simulink model "Optimized_Architecture"  (R2015b)
settings: Solver=FixedStepDiscrete  SolverMode=SingleTasking  StartTime=0.0  StopTime=1000e-6  RelTol=1e-3
libraries: shlslibv1 x282
(part 2 of 2)

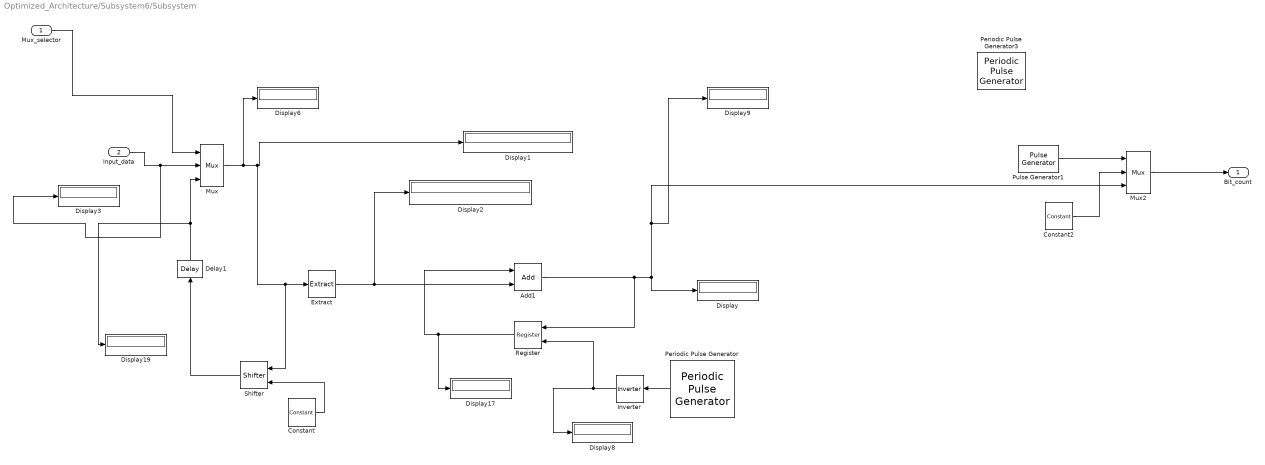
== system Optimized_Architecture/Subsystem6/Subsystem ==
  Mux_selector : Inport
  Input_data : Inport  Port=2
  Add1 : shlslibv1/Math Functions/Add  syn_add_opr=++  syn_out_f=Specify  syn_out_wl=10  syn_out_fl=0  syn_out_dt=unsigned  syn_out_sat=off  syn_out_rnd=Floor (Truncate)  synBlockType=primitive  synLatency=0  synBlockId=96  syn_sum_of_rows=off  syn_inh_port=off  syn_inh_st=on  syn_inh_stf=1  syn_en_pipe=off  syn_pipe_stg=10  syn_flow_ctrl=off
  Constant : shlslibv1/Sources/Constant  syn_cst_val=1  syn_cst_format=Automatic  syn_cst_wl=1  syn_cst_fl=0  syn_cst_dt=unsigned  syn_cst_rnd=on  syn_cst_st=-1  synBlockType=primitive  synLatency=0  synBlockId=15
  Constant2 : shlslibv1/Sources/Constant  syn_cst_val=0  syn_cst_format=Automatic  syn_cst_wl=1  syn_cst_fl=0  syn_cst_dt=unsigned  syn_cst_rnd=on  syn_cst_st=-1  synBlockType=primitive  synLatency=0  synBlockId=15
  Delay1 : shlslibv1/Memories/Delay  syn_delay_val=30  synBlockType=primitive  synLatency=30  synBlockId=104
  Display{,1..3,6,8..9,17,19} (9 alike) : Display
      Display settings: Format=decimal (Stored Integer)
      Display1 settings: Format=binary (Stored Integer)
      Display17 settings: Format=decimal (Stored Integer)
      Display19 settings: Format=decimal (Stored Integer)
      Display2 settings: Format=binary (Stored Integer)
      Display3 settings: Format=decimal (Stored Integer)
      Display8 settings: Format=decimal (Stored Integer)
      Display9 settings: Format=decimal (Stored Integer)
  Extract : shlslibv1/Signal Operations/Extract  syn_extract_vec=0  synBlockType=primitive  synLatency=0  synBlockId=17
  Inverter : shlslibv1/Math Functions/Inverter  syn_out_f=Automatic  syn_out_wl=16  syn_out_fl=8  syn_out_dt=signed  synBlockType=primitive  synLatency=0  synBlockId=10
  Mux : shlslibv1/Signal Operations/Mux  syn_in_nb=2  syn_out_f=Specify  syn_out_wl=10  syn_out_fl=0  syn_out_dt=unsigned  syn_en_se=off  synBlockType=primitive  synLatency=0  synBlockId=16
  Mux2 : shlslibv1/Signal Operations/Mux  syn_in_nb=2  syn_out_f=Specify  syn_out_wl=10  syn_out_fl=0  syn_out_dt=unsigned  syn_en_se=off  synBlockType=primitive  synLatency=0  synBlockId=16
  Periodic Pulse Generator : shlslibv1/Sources/Periodic Pulse  Generator  syn_period_type=Constant  syn_period=309  syn_pw_type=Constant  syn_pw=307  syn_pd_type=Constant  syn_pd=0  syn_en_port=off  syn_st=1/1e6  synBlockType=custom  synLatency=0
  Periodic Pulse Generator3 : shlslibv1/Sources/Periodic Pulse  Generator  syn_period_type=Constant  syn_period=312  syn_pw_type=Constant  syn_pw=31  syn_pd_type=Constant  syn_pd=0  syn_en_port=off  syn_st=1/1e6  synBlockType=custom  synLatency=0
  Pulse Generator1 : shlslibv1/Sources/Pulse Generator  syn_siggentype=Step (0 to 1)  syn_usectl=off  syn_trigedge=rising  syn_triginit=low  syn_stpdel=271  syn_impwidth=1  syn_impdel=1  syn_st=1/1e6  synBlockType=custom  synLatency=0
  Register : shlslibv1/Memories/Register  syn_delay_val=30  syn_rst_val=All zeros  syn_rst_vec=5  syn_rst_port=on  syn_en_port=off  synBlockType=custom  synLatency=30
  Shifter : shlslibv1/Math Functions/Shifter  syn_shifter_opr=>>  syn_out_f=Specify  syn_out_wl=10  syn_out_fl=0  syn_out_dt=unsigned  synBlockType=primitive  synLatency=0  synBlockId=12
  Bit_count : Outport
  wires:
  Add1/1 -> Register/1, Mux2/3, Display9/1, Display/1
  Delay1/1 -> Display19/1, Mux/3
  Constant/1 -> Shifter/2
  Mux_selector/1 -> Mux/1
  Input_data/1 -> Display3/1, Mux/2
  Mux/1 -> Display6/1, Extract/1, Shifter/1, Display1/1
  Periodic Pulse Generator/1 -> Inverter/1
  Register/1 -> Display17/1, Add1/1
  Shifter/1 -> Delay1/1
  Extract/1 -> Display2/1, Add1/2
  Mux2/1 -> Bit_count/1
  Constant2/1 -> Mux2/2
  Inverter/1 -> Register/2, Display8/1
  Pulse Generator1/1 -> Mux2/1

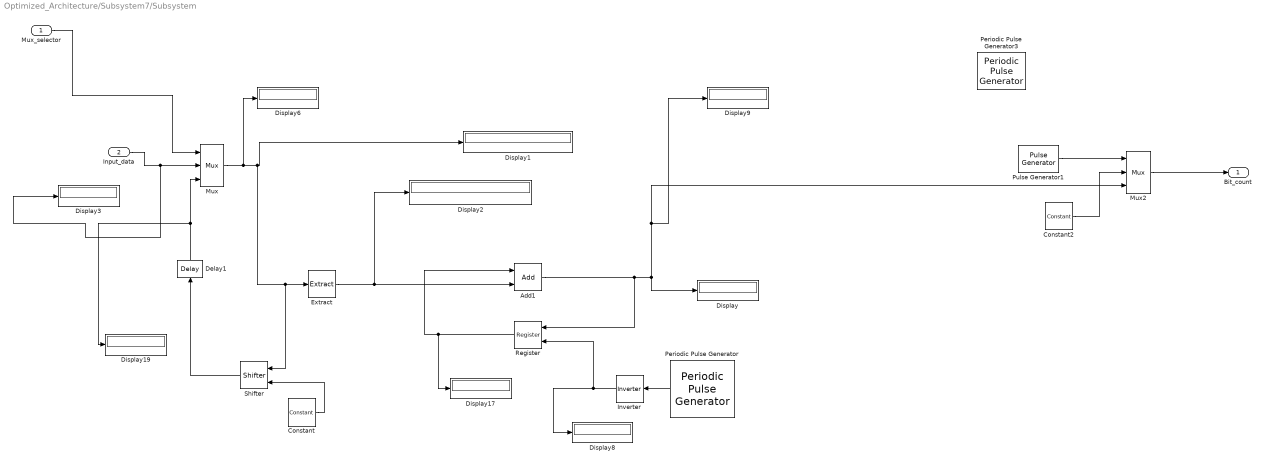
== system Optimized_Architecture/Subsystem7/Subsystem ==
  Mux_selector : Inport
  Input_data : Inport  Port=2
  Add1 : shlslibv1/Math Functions/Add  syn_add_opr=++  syn_out_f=Specify  syn_out_wl=10  syn_out_fl=0  syn_out_dt=unsigned  syn_out_sat=off  syn_out_rnd=Floor (Truncate)  synBlockType=primitive  synLatency=0  synBlockId=96  syn_sum_of_rows=off  syn_inh_port=off  syn_inh_st=on  syn_inh_stf=1  syn_en_pipe=off  syn_pipe_stg=10  syn_flow_ctrl=off
  Constant : shlslibv1/Sources/Constant  syn_cst_val=1  syn_cst_format=Automatic  syn_cst_wl=1  syn_cst_fl=0  syn_cst_dt=unsigned  syn_cst_rnd=on  syn_cst_st=-1  synBlockType=primitive  synLatency=0  synBlockId=15
  Constant2 : shlslibv1/Sources/Constant  syn_cst_val=0  syn_cst_format=Automatic  syn_cst_wl=1  syn_cst_fl=0  syn_cst_dt=unsigned  syn_cst_rnd=on  syn_cst_st=-1  synBlockType=primitive  synLatency=0  synBlockId=15
  Delay1 : shlslibv1/Memories/Delay  syn_delay_val=30  synBlockType=primitive  synLatency=30  synBlockId=104
  Display{,1..3,6,8..9,17,19} (9 alike) : Display
      Display settings: Format=decimal (Stored Integer)
      Display1 settings: Format=binary (Stored Integer)
      Display17 settings: Format=decimal (Stored Integer)
      Display19 settings: Format=decimal (Stored Integer)
      Display2 settings: Format=binary (Stored Integer)
      Display3 settings: Format=decimal (Stored Integer)
      Display8 settings: Format=decimal (Stored Integer)
      Display9 settings: Format=decimal (Stored Integer)
  Extract : shlslibv1/Signal Operations/Extract  syn_extract_vec=0  synBlockType=primitive  synLatency=0  synBlockId=17
  Inverter : shlslibv1/Math Functions/Inverter  syn_out_f=Automatic  syn_out_wl=16  syn_out_fl=8  syn_out_dt=signed  synBlockType=primitive  synLatency=0  synBlockId=10
  Mux : shlslibv1/Signal Operations/Mux  syn_in_nb=2  syn_out_f=Specify  syn_out_wl=10  syn_out_fl=0  syn_out_dt=unsigned  syn_en_se=off  synBlockType=primitive  synLatency=0  synBlockId=16
  Mux2 : shlslibv1/Signal Operations/Mux  syn_in_nb=2  syn_out_f=Specify  syn_out_wl=10  syn_out_fl=0  syn_out_dt=unsigned  syn_en_se=off  synBlockType=primitive  synLatency=0  synBlockId=16
  Periodic Pulse Generator : shlslibv1/Sources/Periodic Pulse  Generator  syn_period_type=Constant  syn_period=309  syn_pw_type=Constant  syn_pw=307  syn_pd_type=Constant  syn_pd=0  syn_en_port=off  syn_st=1/1e6  synBlockType=custom  synLatency=0
  Periodic Pulse Generator3 : shlslibv1/Sources/Periodic Pulse  Generator  syn_period_type=Constant  syn_period=312  syn_pw_type=Constant  syn_pw=31  syn_pd_type=Constant  syn_pd=0  syn_en_port=off  syn_st=1/1e6  synBlockType=custom  synLatency=0
  Pulse Generator1 : shlslibv1/Sources/Pulse Generator  syn_siggentype=Step (0 to 1)  syn_usectl=off  syn_trigedge=rising  syn_triginit=low  syn_stpdel=271  syn_impwidth=1  syn_impdel=1  syn_st=1/1e6  synBlockType=custom  synLatency=0
  Register : shlslibv1/Memories/Register  syn_delay_val=30  syn_rst_val=All zeros  syn_rst_vec=5  syn_rst_port=on  syn_en_port=off  synBlockType=custom  synLatency=30
  Shifter : shlslibv1/Math Functions/Shifter  syn_shifter_opr=>>  syn_out_f=Specify  syn_out_wl=10  syn_out_fl=0  syn_out_dt=unsigned  synBlockType=primitive  synLatency=0  synBlockId=12
  Bit_count : Outport
  wires:
  Add1/1 -> Register/1, Mux2/3, Display9/1, Display/1
  Delay1/1 -> Display19/1, Mux/3
  Constant/1 -> Shifter/2
  Mux_selector/1 -> Mux/1
  Input_data/1 -> Display3/1, Mux/2
  Mux/1 -> Display6/1, Extract/1, Shifter/1, Display1/1
  Periodic Pulse Generator/1 -> Inverter/1
  Register/1 -> Display17/1, Add1/1
  Shifter/1 -> Delay1/1
  Extract/1 -> Display2/1, Add1/2
  Mux2/1 -> Bit_count/1
  Constant2/1 -> Mux2/2
  Inverter/1 -> Register/2, Display8/1
  Pulse Generator1/1 -> Mux2/1

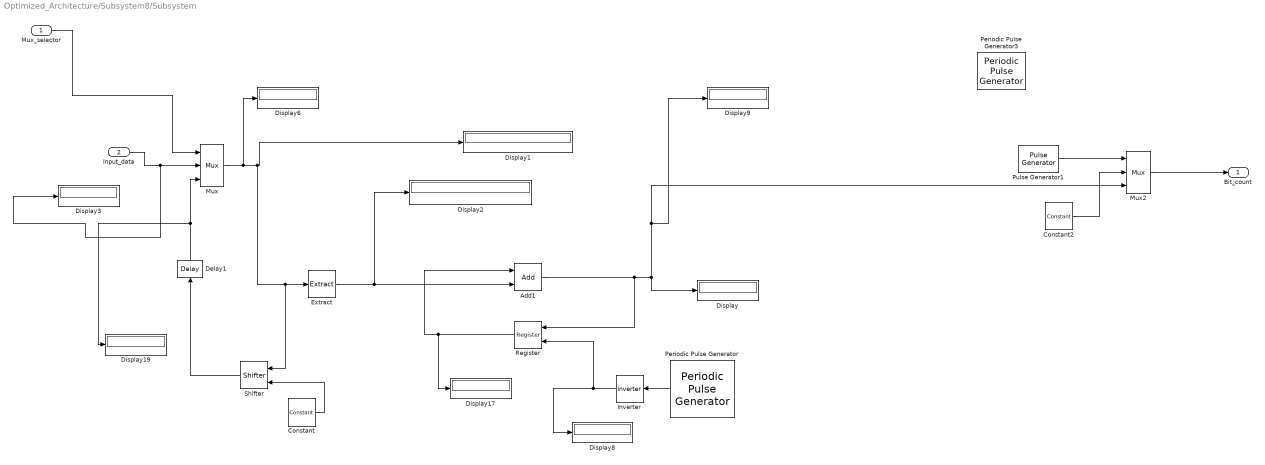
== system Optimized_Architecture/Subsystem8/Subsystem ==
  Mux_selector : Inport
  Input_data : Inport  Port=2
  Add1 : shlslibv1/Math Functions/Add  syn_add_opr=++  syn_out_f=Specify  syn_out_wl=10  syn_out_fl=0  syn_out_dt=unsigned  syn_out_sat=off  syn_out_rnd=Floor (Truncate)  synBlockType=primitive  synLatency=0  synBlockId=96  syn_sum_of_rows=off  syn_inh_port=off  syn_inh_st=on  syn_inh_stf=1  syn_en_pipe=off  syn_pipe_stg=10  syn_flow_ctrl=off
  Constant : shlslibv1/Sources/Constant  syn_cst_val=1  syn_cst_format=Automatic  syn_cst_wl=1  syn_cst_fl=0  syn_cst_dt=unsigned  syn_cst_rnd=on  syn_cst_st=-1  synBlockType=primitive  synLatency=0  synBlockId=15
  Constant2 : shlslibv1/Sources/Constant  syn_cst_val=0  syn_cst_format=Automatic  syn_cst_wl=1  syn_cst_fl=0  syn_cst_dt=unsigned  syn_cst_rnd=on  syn_cst_st=-1  synBlockType=primitive  synLatency=0  synBlockId=15
  Delay1 : shlslibv1/Memories/Delay  syn_delay_val=30  synBlockType=primitive  synLatency=30  synBlockId=104
  Display{,1..3,6,8..9,17,19} (9 alike) : Display
      Display settings: Format=decimal (Stored Integer)
      Display1 settings: Format=binary (Stored Integer)
      Display17 settings: Format=decimal (Stored Integer)
      Display19 settings: Format=decimal (Stored Integer)
      Display2 settings: Format=binary (Stored Integer)
      Display3 settings: Format=decimal (Stored Integer)
      Display8 settings: Format=decimal (Stored Integer)
      Display9 settings: Format=decimal (Stored Integer)
  Extract : shlslibv1/Signal Operations/Extract  syn_extract_vec=0  synBlockType=primitive  synLatency=0  synBlockId=17
  Inverter : shlslibv1/Math Functions/Inverter  syn_out_f=Automatic  syn_out_wl=16  syn_out_fl=8  syn_out_dt=signed  synBlockType=primitive  synLatency=0  synBlockId=10
  Mux : shlslibv1/Signal Operations/Mux  syn_in_nb=2  syn_out_f=Specify  syn_out_wl=10  syn_out_fl=0  syn_out_dt=unsigned  syn_en_se=off  synBlockType=primitive  synLatency=0  synBlockId=16
  Mux2 : shlslibv1/Signal Operations/Mux  syn_in_nb=2  syn_out_f=Specify  syn_out_wl=10  syn_out_fl=0  syn_out_dt=unsigned  syn_en_se=off  synBlockType=primitive  synLatency=0  synBlockId=16
  Periodic Pulse Generator : shlslibv1/Sources/Periodic Pulse  Generator  syn_period_type=Constant  syn_period=309  syn_pw_type=Constant  syn_pw=307  syn_pd_type=Constant  syn_pd=0  syn_en_port=off  syn_st=1/1e6  synBlockType=custom  synLatency=0
  Periodic Pulse Generator3 : shlslibv1/Sources/Periodic Pulse  Generator  syn_period_type=Constant  syn_period=312  syn_pw_type=Constant  syn_pw=31  syn_pd_type=Constant  syn_pd=0  syn_en_port=off  syn_st=1/1e6  synBlockType=custom  synLatency=0
  Pulse Generator1 : shlslibv1/Sources/Pulse Generator  syn_siggentype=Step (0 to 1)  syn_usectl=off  syn_trigedge=rising  syn_triginit=low  syn_stpdel=271  syn_impwidth=1  syn_impdel=1  syn_st=1/1e6  synBlockType=custom  synLatency=0
  Register : shlslibv1/Memories/Register  syn_delay_val=30  syn_rst_val=All zeros  syn_rst_vec=5  syn_rst_port=on  syn_en_port=off  synBlockType=custom  synLatency=30
  Shifter : shlslibv1/Math Functions/Shifter  syn_shifter_opr=>>  syn_out_f=Specify  syn_out_wl=10  syn_out_fl=0  syn_out_dt=unsigned  synBlockType=primitive  synLatency=0  synBlockId=12
  Bit_count : Outport
  wires:
  Add1/1 -> Register/1, Mux2/3, Display9/1, Display/1
  Delay1/1 -> Display19/1, Mux/3
  Constant/1 -> Shifter/2
  Mux_selector/1 -> Mux/1
  Input_data/1 -> Display3/1, Mux/2
  Mux/1 -> Display6/1, Extract/1, Shifter/1, Display1/1
  Periodic Pulse Generator/1 -> Inverter/1
  Register/1 -> Display17/1, Add1/1
  Shifter/1 -> Delay1/1
  Extract/1 -> Display2/1, Add1/2
  Mux2/1 -> Bit_count/1
  Constant2/1 -> Mux2/2
  Inverter/1 -> Register/2, Display8/1
  Pulse Generator1/1 -> Mux2/1
